simulink model "LAB_C1"  (R2021b)
settings: Solver=FixedStepAuto  StartTime=0.0  StopTime=5e-6  FixedStep=5e-8  RelTol=1e-3
undefined symbols (not defined in the file or in its folder): xc7k160tfbg676
libraries: hdlBasic x22, vmcUtilities x1
settings Model: Creator=15145  LastModifiedBy=Abdel
settings DataIOCC: ReturnWorkspaceOutputs=off

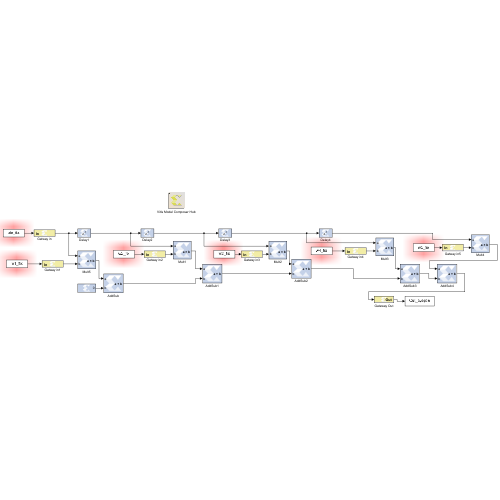
[thumbnail: Simulink's stored preview of the top-level diagram]
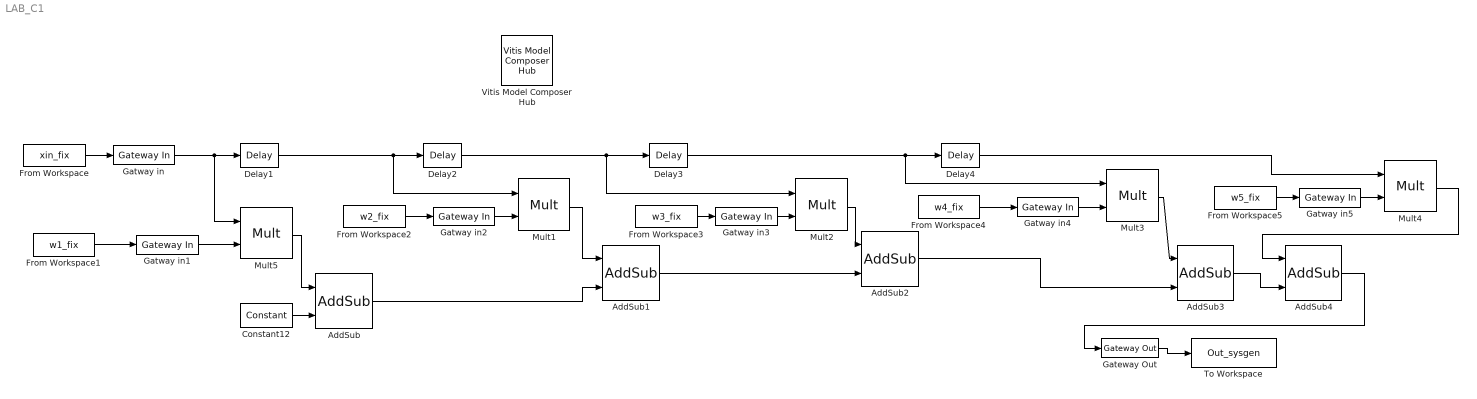
== system LAB_C1 ==
  AddSub{,1..4} (5 alike) : hdlBasic/AddSub  mode=Addition  use_carryin=off  use_carryout=off  en=off  latency=0  precision=Full  arith_type=Unsigned  n_bits=16  bin_pt=14  quantization=Truncate  overflow=Wrap  use_behavioral_HDL=off  hw_selection=Fabric  pipelined=off  XmcBlockStatus=1  maskContainerNames=tabcontainer1  block_type=addsub  block_config=sysgen:Addsub_config
  Constant12 : hdlBasic/Constant  const=0  gui_display_data_type=Fixed-point  arith_type=Unsigned  n_bits=8  bin_pt=0  preci_type=Single  exp_width=8  frac_width=24  explicit_period=on  period=5e-8  XmcBlockStatus=1  maskContainerNames=tabcontainer1  block_type=constant  block_config=sysgen:Constant_config
  Delay{1..4} (4 alike) : hdlBasic/Delay  rst=off  en=off  latency=1  reg_retiming=off  XmcBlockStatus=1  maskContainerNames=group1  block_type=delay  block_config=sysgen:Delay_config
  From Workspace : FromWorkspace  VariableName=xin_fix  SampleTime=5e-8  Interpolate=off  OutputAfterFinalValue=Holding final value
  From Workspace1 : FromWorkspace  VariableName=w1_fix  SampleTime=5e-8  Interpolate=off  OutputAfterFinalValue=Holding final value
  From Workspace2 : FromWorkspace  VariableName=w2_fix  SampleTime=5e-8  Interpolate=off  OutputAfterFinalValue=Holding final value
  From Workspace3 : FromWorkspace  VariableName=w3_fix  SampleTime=5e-8  Interpolate=off  OutputAfterFinalValue=Holding final value
  From Workspace4 : FromWorkspace  VariableName=w4_fix  SampleTime=5e-8  Interpolate=off  OutputAfterFinalValue=Holding final value
  From Workspace5 : FromWorkspace  VariableName=w5_fix  SampleTime=5e-8  Interpolate=off  OutputAfterFinalValue=Holding final value
  Gateway Out : hdlBasic/Gateway Out  inherit_from_input=off  hdl_port=on  rows=1  columns=1  UseAsDAC=off  DACChannel='1'  interface=None  automatic_assignment=on  address_offset=hex2dec('00')  intf_name=''  intf_description=''  timing_constraint=None  locs_specified=off  LOCs={}  io_standard={}  XmcBlockStatus=1  maskContainerNames=group4  block_type=gatewayout  block_config=sysgen:gateway_out_config  block_width_w=590  block_height_w=620  block_width=620  block_height=750
  Gatway in{,1..5} (6 alike) : hdlBasic/Gateway In  gui_display_data_type=Fixed-point  arith_type=Signed (2's comp)  n_bits=16  bin_pt=15  preci_type=Single  exp_width=8  frac_width=24  rows=1  columns=1  quantization="Round  (unbiased: +/- Inf)"  overflow=Saturate  period=1/20e6  UseAsADC=off  ADCChannel='1'  interface=None  automatic_assignment=on  address_offset=hex2dec('00')  intf_name=''  intf_description=''  default_value=0  timing_constraint=None  locs_specified=off  LOCs={}  io_standard={}  inherit_from_input=off  hdl_port=on  XmcBlockStatus=1  maskContainerNames=group4  block_type=gatewayin  block_config=sysgen:gateway_in_config  block_width_w=590  block_height_w=620  block_width=640  block_height=850
  Mult{1..5} (5 alike) : hdlBasic/Mult  precision=User Defined  arith_type="Signed  (2's comp)"  n_bits=32  bin_pt=16  quantization=Truncate  overflow=Wrap  en=off  latency=0  use_behavioral_HDL=off  opt=Speed  use_embedded=on  optimum_pipeline=off  pipeline=on  use_rpm=on  placement_style=Triangular  XmcBlockStatus=1  maskContainerNames=group1  block_type=mult  block_config=sysgen:Mult_config
  To Workspace : ToWorkspace  VariableName=Out_sysgen  SampleTime=5e-8
  Vitis Model Composer Hub : vmcUtilities/Vitis Model Composer Hub  Tag=genX  CodeGeneration=off  SubsystemName=<enter or select subsystem name>  TargetDirectory=./code  ExportType=HLS C++ code  IpVendor=xilinx.com  IpLibrary=hls  IpVersion=1.0  IpHWLanguage=Verilog  AieCompilerOptions={}  CreateTestbench=off  TestbenchStackSize=10  RunAieSim=off  AieSimTimeout=50000  RunAieSimProfiling=off  LaunchVitisAnalyzer=off  PlotOutput=off  RunX86Sim=off  X86SimTimeout=10  GenHwImage=off  PlatformType=Not Specified  HwSystemType=Baremetal  HwValidationTarget=hw  ProjDevice=xc7k160tfbg676-3  ProjDevicePart=xc7k160tfbg676-3  SamplePeriod=-1  ClockFrequency=200  DataPathParallelism=1  xilinxfamily=kintex7  part=xc7k160t  speed=-3  package=fbg676  directory=./netlist  testbench=off  incr_netlist=off  synthesis_tool=Vivado  clock_wrapper=Clock Enables  dbl_ovrd=According to Block Masks  dcm_input_clock_period=10  sysclk_period=10  simulink_period=10e-9  eval_field=0
  wires:
  Gatway in/1 -> Mult5/1, Delay1/1
  Gatway in1/1 -> Mult5/2
  Constant12/1 -> AddSub/2
  Mult5/1 -> AddSub/1
  From Workspace1/1 -> Gatway in1/1
  From Workspace/1 -> Gatway in/1
  From Workspace2/1 -> Gatway in2/1
  Gatway in2/1 -> Mult1/2
  Delay1/1 -> Mult1/1, Delay2/1
  Mult1/1 -> AddSub1/1
  AddSub/1 -> AddSub1/2
  Gatway in3/1 -> Mult2/2
  From Workspace3/1 -> Gatway in3/1
  Mult2/1 -> AddSub2/1
  Delay2/1 -> Delay3/1, Mult2/1
  AddSub1/1 -> AddSub2/2
  Gatway in4/1 -> Mult3/2
  From Workspace4/1 -> Gatway in4/1
  Delay3/1 -> Mult3/1, Delay4/1
  Mult3/1 -> AddSub3/1
  AddSub2/1 -> AddSub3/2
  Gatway in5/1 -> Mult4/2
  From Workspace5/1 -> Gatway in5/1
  Mult4/1 -> AddSub4/1
  Delay4/1 -> Mult4/1
  AddSub3/1 -> AddSub4/2
  AddSub4/1 -> Gateway Out/1
  Gateway Out/1 -> To Workspace/1
